simulink model "RevisedStraightLine2"  (R2015b)
settings: Solver=FixedStepAuto  StartTime=0.0  StopTime=1000  FixedStep=0.001  RelTol=1e-7
values from neighbouring files (symbols this model uses):
  aa = a(i)    [BeardMethod.m]
  alpha = 1.65    [BeardMethod.m]    (also in OrbitCenter.m = abs((ang1-ang2)/2); RevisedMethod.m)
  ang = angle(i)    [BeardMethod.m]    (also in RevisedMethod.m = 0)
  bb = b(i)    [BeardMethod.m]
  chi_inf = pi/2    (= 1.57079632679)    [BeardMethod.m]    (also in RevisedMethod.m)
  course_int = course_int+2*pi    (= 6.28318530718)    [BeardMethod.m]    (also in RevisedMethod.m = -0.785398163397)
  endx = E2(1)-6    [BeardMethod.m]    (also in RevisedMethod.m = 300)
  epsi = 0.1    [BeardMethod.m]    (also in RevisedMethod.m = 0.5)
  i = 1    [BeardMethod.m]    (also in RevisedMethod.m = 1, go left, x decreases))
  k = 0.02    [BeardMethod.m]    (also in RevisedMethod.m = 0.1)
  kk = pi/2    (= 1.57079632679)    [BeardMethod.m]    (also in RevisedMethod.m)
  phiw = 230/180*pi    (= 4.01425727959)    [BeardMethod.m]    (also in RevisedMethod.m)
  Va = 13    [BeardMethod.m]    (also in RevisedMethod.m)
  W = 6    [RevisedMethod.m]
  x_int = x.data(end)    [BeardMethod.m]    (also in RevisedMethod.m = 0)
  y_int = y.data(end)    [BeardMethod.m]    (also in RevisedMethod.m = 80)
libraries: simulink x1
settings Model: Creator=Bingyu Zhou  LastModifiedBy=Bingyu Zhou

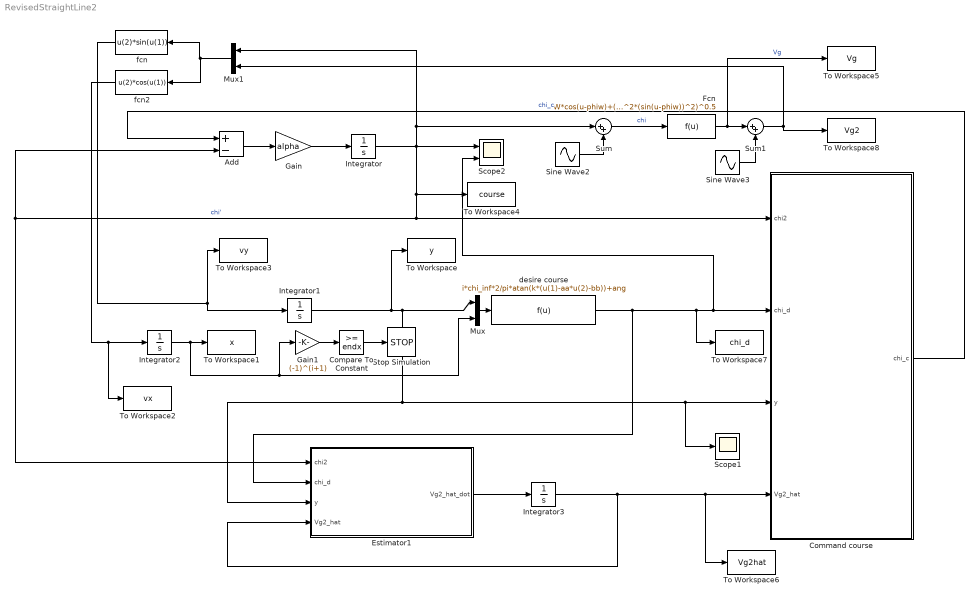
== system RevisedStraightLine2 ==
  Add : Sum  Inputs=+-
  Command course : Subsystem
  Compare To Constant : simulink/Logic and Bit Operations/Compare To Constant  relop=>=  const=endx  OutDataTypeStr=boolean
  Estimator1 : MATLAB Function  TreatAsAtomicUnit=on
  Fcn : Fcn  Expr=W*cos(u-phiw)+(Va^2-W^2*(sin(u-phiw))^2)^0.5
  Gain : Gain  Gain=alpha
  Gain1 : Gain  Gain=(-1)^(i+1)
  Integrator : Integrator  InitialCondition=course_int
  Integrator1 : Integrator  InitialCondition=y_int
  Integrator2 : Integrator  InitialCondition=x_int
  Integrator3 : Integrator  InitialCondition=12.1
  Mux : Mux  Inputs=2
  Mux1 : Mux  Inputs=2
  Scope1 : Scope
  Scope2 : Scope  NumInputPorts=2
  Sine Wave2 : Sin  Amplitude=0.2  Frequency=0.5  SampleTime=0
  Sine Wave3 : Sin  Frequency=0.5  SampleTime=0
  Stop Simulation : Stop
  Sum : Sum  Inputs=|++
  Sum1 : Sum  Inputs=|++
  To Workspace : ToWorkspace  VariableName=y  SaveFormat=Timeseries  SampleTime=-1
  To Workspace1 : ToWorkspace  VariableName=x  SaveFormat=Timeseries  SampleTime=-1
  To Workspace2 : ToWorkspace  VariableName=vx  SaveFormat=Timeseries  SampleTime=-1
  To Workspace3 : ToWorkspace  VariableName=vy  SaveFormat=Timeseries  SampleTime=-1
  To Workspace4 : ToWorkspace  VariableName=course  SaveFormat=Timeseries  SampleTime=-1
  To Workspace5 : ToWorkspace  VariableName=Vg  SaveFormat=Timeseries  SampleTime=-1
  To Workspace6 : ToWorkspace  VariableName=Vg2hat  SaveFormat=Timeseries  SampleTime=-1
  To Workspace7 : ToWorkspace  VariableName=chi_d  SaveFormat=Timeseries  SampleTime=-1
  To Workspace8 : ToWorkspace  VariableName=Vg2  SaveFormat=Timeseries  SampleTime=-1
  desire course : Fcn  Expr=i*chi_inf*2/pi*atan(k*(u(1)-aa*u(2)-bb))+ang
  fcn : Fcn  Expr=u(2)*sin(u(1))
  fcn2 : Fcn  Expr=u(2)*cos(u(1))
  wires:
  Add/1 -> Gain/1
  Gain/1 -> Integrator/1
  Integrator/1 -> Mux1/1, Sum/1, Scope2/1, To Workspace4/1, Command course/1(chi2), Add/2, Estimator1/1(chi2)  "chi'"
  Integrator1/1 -> To Workspace/1, Mux/1, Estimator1/3(y), Scope1/1, Command course/3(y)
  desire course/1 -> Estimator1/2(chi_d), To Workspace7/1, Scope2/2, Command course/2(chi_d)
  Command course/1(chi_c) -> Add/1  "chi_c"
  Integrator2/1 -> Gain1/1, Mux/2, To Workspace1/1
  Estimator1/1(Vg2_hat_dot) -> Integrator3/1
  Integrator3/1 -> Estimator1/4(Vg2_hat), Command course/4(Vg2_hat), To Workspace6/1
  fcn/1 -> Integrator1/1, To Workspace3/1
  fcn2/1 -> To Workspace2/1, Integrator2/1
  Mux/1 -> desire course/1
  Compare To Constant/1 -> Stop Simulation/1
  Gain1/1 -> Compare To Constant/1
  Sine Wave2/1 -> Sum/2
  Sum/1 -> Fcn/1  "chi"
  Fcn/1 -> To Workspace5/1, Sum1/1  "Vg"
  Sine Wave3/1 -> Sum1/2
  Sum1/1 -> Mux1/2, To Workspace8/1
  Mux1/1 -> fcn2/1, fcn/1

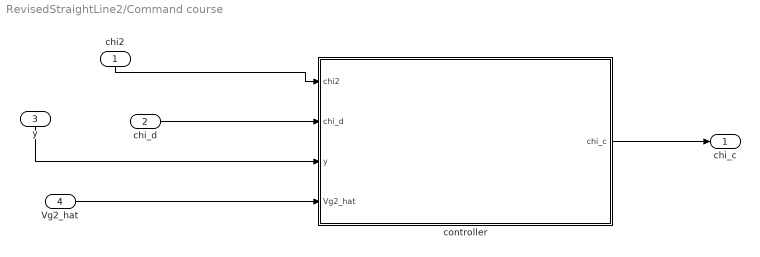
== system RevisedStraightLine2/Command course ==
  chi2 : Inport
  chi_d : Inport  Port=2
  y : Inport  Port=3
  Vg2_hat : Inport  Port=4
  controller : MATLAB Function  TreatAsAtomicUnit=on
  chi_c : Outport
  wires:
  chi_d/1 -> controller/2(chi_d)
  controller/1(chi_c) -> chi_c/1
  chi2/1 -> controller/1(chi2)
  y/1 -> controller/3(y)
  Vg2_hat/1 -> controller/4(Vg2_hat)

== matlab function RevisedStraightLine2/Command course/controller ==
  data: chi2 input; chi_d input; y input; Vg2_hat input; chi_c output; epsi parameter; chi_inf parameter; k parameter; kk parameter; alpha parameter
function chi_c = CommandCourse(chi2,chi_d,y,Vg2_hat,epsi,chi_inf,k,kk,alpha)
%generate command course angle chi_c
term =(chi2-chi_d)/epsi;
if abs(term)<=1
    sat=term;
else
    sat=sign(term);
end

chi_c=chi2-chi_inf*2/pi/alpha*k/(1+(k*y)^2)*Vg2_hat*sin(chi2)-kk/alpha*sat;


end

== matlab function RevisedStraightLine2/Estimator1 ==
  data: chi2 input; chi_d input; y input; Vg2_hat input; Vg2_hat_dot output; y_int parameter; W parameter; Va parameter; epsi parameter; phiw parameter; chi_inf parameter; k parameter; kk parameter
function Vg2_hat_dot = estimator(chi2,chi_d,y,Vg2_hat,y_int,W,Va,epsi,phiw,chi_inf,k,kk)
%estimator of Vg'
Gamma = 0.5;
rho = y_int^2/pi^2; %positive scale factor used to weight the terms so that y and chi are similar in magnitude

diff_chi = chi2-chi_d; % error of course angle

term =diff_chi/epsi;
if abs(term)<=1
    sat=term;
else
    sat=sign(term);
end
% derivative of Vg' over x'
der = W*sin(phiw-chi2)+(Va^2-W^2*(sin(phiw-chi2))^2)^(-0.5)*W^2*sin(phiw-chi2)*cos(phiw-chi2); % partial derivative of Vg' over chi'

Vg2_hat_dot = Gamma*rho*diff_chi*chi_inf*2/pi*k/(1+(k*y)^2)*sin(chi2)-der*(chi_inf*2/pi*k/(1+(k*y)^2)*Vg2_hat*sin(chi2)+kk*sat);

end
